simulink model "position_control_model"  (R2018b)
settings: Solver=VariableStepAuto  StartTime=0.0  StopTime=10.0  RelTol=1e-3
values from neighbouring files (symbols this model uses):
  a = 100    [PID_control_design_of_DC_motor.m]
  GP_den = [1 1021 4845 0]    [PID_control_design_of_DC_motor.m]
  GP_num = [46163]    [PID_control_design_of_DC_motor.m]
  KD = 0.0895    [PID_control_design_of_DC_motor.m]
  KI = 1.4006    [PID_control_design_of_DC_motor.m]
  KP = 0.7044    [PID_control_design_of_DC_motor.m]
settings Model: Creator=Christopher  LastModifiedBy=chris

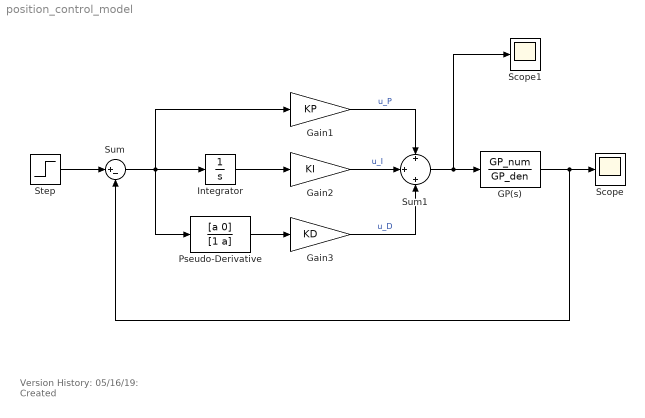
== system position_control_model ==
  note: Version History:
      | 05/16/19: Created
  GP(s) : TransferFcn  Numerator=GP_num  Denominator=GP_den
  Gain1 : Gain  Gain=KP
  Gain2 : Gain  Gain=KI
  Gain3 : Gain  Gain=KD
  Integrator : Integrator
  Pseudo-Derivative : TransferFcn  Numerator=[a 0]  Denominator=[1 a]
  Scope : Scope
  Scope1 : Scope
  Step : Step  SampleTime=0
  Sum : Sum  Inputs=|+-
  Sum1 : Sum  Inputs=+|+|+
  wires:
  Step/1 -> Sum/1
  Sum/1 -> Pseudo-Derivative/1, Integrator/1, Gain1/1
  Gain1/1 -> Sum1/1  "u_P"
  Integrator/1 -> Gain2/1
  Sum1/1 -> Scope1/1, GP(s)/1
  Gain2/1 -> Sum1/2  "u_I"
  Pseudo-Derivative/1 -> Gain3/1
  Gain3/1 -> Sum1/3  "u_D"
  GP(s)/1 -> Sum/2, Scope/1
